simulink library "orbitProp2B_sl"  (R2023b)
settings: Solver=VariableStepAuto  StartTime=0.0  StopTime=10.0  RelTol=1e-3
undefined symbols (not defined in the file): mu, satPosition0, satVelocity0
settings Model: Creator=gilbu  LastModifiedBy=gilbu
settings ModelReferenceCC: EnableRefExpFcnMdlSchedulingChecks=on

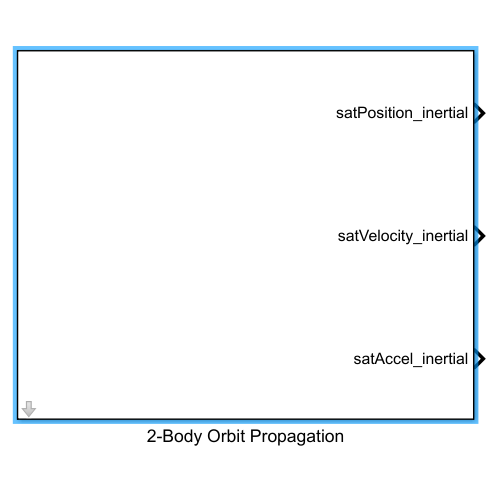
[thumbnail: Simulink's stored preview of the top-level diagram]
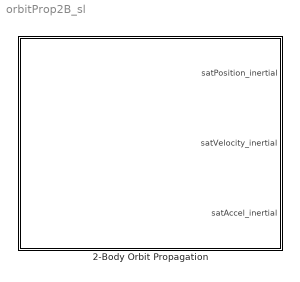
== system orbitProp2B_sl ==
  2-Body Orbit Propagation : Subsystem  mask{mu=mu, satPosition0=satPosition0, satVelocity0=satVelocity0}
      mask prompts: mu "Graviational Parameter [m3/s2] <3>"; satPosition0 "Initial Satellite Position [m]  <3>"; satVelocity0 "Initial Satellite Velocity [m/s] <3>"
      mask DialogControl DescTextVar Prompt: Two-body Orbit Dynamics. Given gravitaitonal parameter, initial position and velocity propagate orbit for given time.

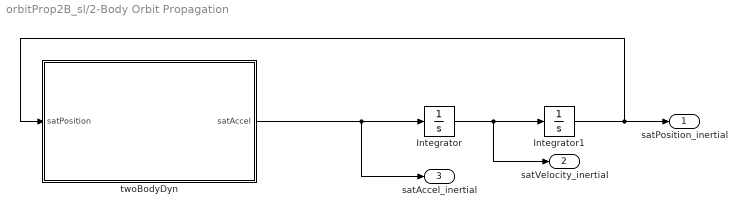
== system orbitProp2B_sl/2-Body Orbit Propagation ==
  Integrator : Integrator  InitialCondition=satVelocity0
  Integrator1 : Integrator  InitialCondition=satPosition0
  twoBodyDyn : MATLAB Function  TreatAsAtomicUnit=on
  satPosition_inertial : Outport
  satVelocity_inertial : Outport  Port=2
  satAccel_inertial : Outport  Port=3
  wires:
  Integrator1/1 -> satPosition_inertial/1, twoBodyDyn/1(satPosition)
  Integrator/1 -> satVelocity_inertial/1, Integrator1/1
  twoBodyDyn/1(satAccel) -> satAccel_inertial/1, Integrator/1

== matlab function orbitProp2B_sl/2-Body Orbit Propagation/twoBodyDyn ==
  data: satPosition input size=3; satAccel output size=3; mu parameter size=1
function satAccel = twoBodyDyn(satPosition, ...
    mu ... % Parameters
    )
%-------------------------------------------------------------------------------

r = norm(satPosition);

satAccel = -mu/r^3 .* satPosition;
